simulink model "FaceDetectResponseApp"  (R2023a)
settings: Solver=FixedStepAuto  StartTime=0.0  StopTime=inf  RelTol=1e-3
undefined symbols (not defined in the file): Rec, SDTV
libraries: androiduilib x6, visionconversions x3, androidaudiovideolib x2, visiontextngfix x2, androidcommunicationlib x1
settings Model: Creator=The MathWorks, Inc.  LastModifiedBy=aqeel
settings SolverCC: AlgebraicLoopSolver=TrustRegion
settings DataIOCC: ReturnWorkspaceOutputs=off
settings OptimizationCC: EnhancedBackFolding=on  PassReuseOutputArgsAs=Individual arguments  ZeroExternalMemoryAtStartup=off  ZeroInternalMemoryAtStartup=off  MaxStackSize=64  OptimizeBlockOrder=speed  DifferentSizesBufferReuse=on  OptimizationCustomize=off  EfficientTunableParamExpr=on
settings DebuggingCC: ParameterTunabilityLossMsg=error  UnconnectedInputMsg=warning  UnconnectedOutputMsg=warning  UnconnectedLineMsg=warning  ArithmeticOperatorsInVariantConditions=warning
settings HardwareCC: ProdBitPerPointer=32  ProdBitPerSizeT=32  ProdBitPerPtrDiffT=32  ProdLargestAtomicInteger=Long  ProdLargestAtomicFloat=Double  ProdWordSize=32  ProdHWDeviceType=ARM Compatible->ARM Cortex  UseEmbeddedCoderFeatures=off  UseSimulinkCoderFeatures=off
settings ModelReferenceCC: EnableRefExpFcnMdlSchedulingChecks=on
settings SFSimCC: CustomCodeUndefinedFunction=UseInterfaceOnly
settings RTWCC: Description=Embedded Coder  SystemTargetFile=ert.tlc  HardwareBoard=Android Device  TLCOptions="-aInlineSetEventsForThisBaseRateFcn=TLC_FALSE -aSuppressMultiTaskScheduler=TLC_FALSE  -aRateBasedStepFcn=0"  TemplateMakefile=ert_default_tmf  GenerateReport=on  RTWVerbose=off  Toolchain=Android SDK/NDK Tools  LaunchReport=on  DLArmComputeVersion=19.05
settings CodeAppCC: ForceParamTrailComments=on  IgnoreCustomStorageClasses=off  OperatorAnnotations=on  SimulinkDataObjDesc=on  SFDataObjDesc=on  InsertBlockDesc=on
settings ERTTargetCC: SupportNonInlinedSFcns=on

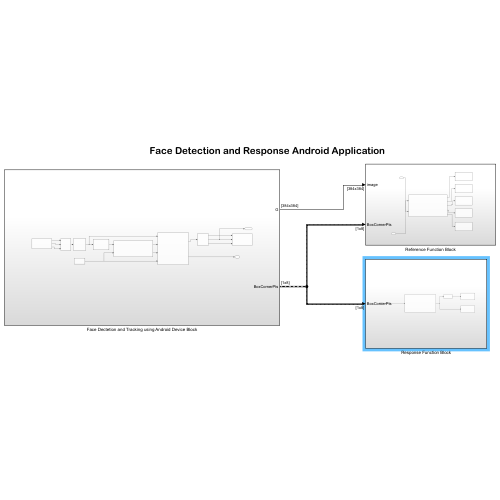
[thumbnail: Simulink's stored preview of the top-level diagram]
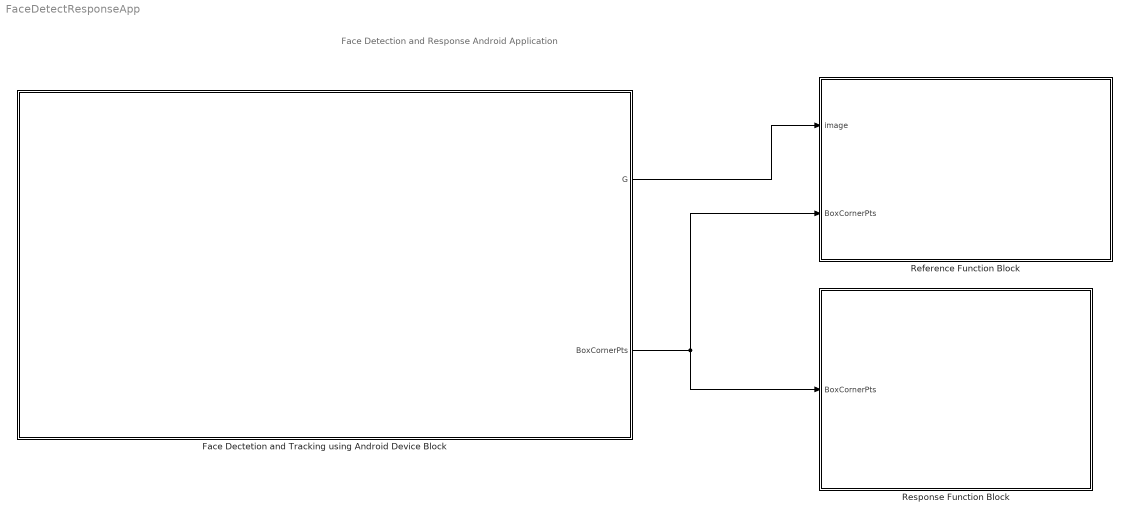
== system FaceDetectResponseApp ==
  note: Face Detection and Response Android Application
  Face Dectetion and Tracking using Android Device Block : Subsystem
  Reference Function Block : Subsystem
  Response Function Block : Subsystem
  wires:
  Face Dectetion and Tracking using Android Device Block/2(BoxCornerPts) -> Response Function Block/1(BoxCornerPts), Reference Function Block/2(BoxCornerPts)
  Face Dectetion and Tracking using Android Device Block/1(G) -> Reference Function Block/1(image)

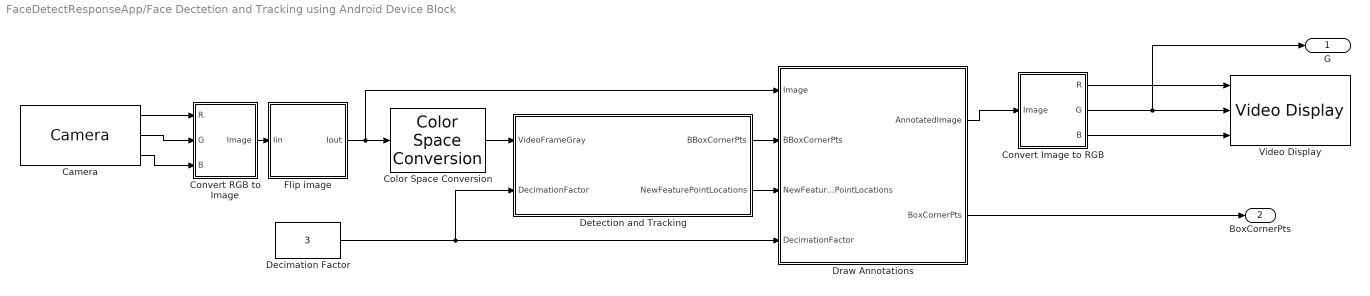
== system FaceDetectResponseApp/Face Dectetion and Tracking using Android Device Block ==
  Camera : androidaudiovideolib/Camera  CameraLocation=Back  CameraResolutions=Back - 384x384  Width=384  Height=384  SampleTime=0.01  BlockPlatform=Android
  Color Space Conversion : visionconversions/Color Space  Conversion  conversion=Obsolete  conversionActive=R'G'B' to intensity  wp_str=D65  rec=Rec. 601 (SDTV)  sys=1125/60/2:1  imagePorts=One multidimensional signal
  Convert Image to RGB : Subsystem
  Convert RGB to Image : Subsystem
  Decimation Factor : Constant  Value=3
  Detection and Tracking : Subsystem
  Draw Annotations : Subsystem
  Flip image : MATLAB Function  TreatAsAtomicUnit=on
  Video Display : androidaudiovideolib/Video Display  BlockPlatform=Android
  G : Outport
  BoxCornerPts : Outport  Port=2
  wires:
  Draw Annotations/2(BoxCornerPts) -> BoxCornerPts/1
  Flip image/1(Iout) -> Draw Annotations/1(Image), Color Space Conversion/1
  Detection and Tracking/1(BBoxCornerPts) -> Draw Annotations/2(BBoxCornerPts)
  Decimation Factor/1 -> Draw Annotations/4(DecimationFactor), Detection and Tracking/2(DecimationFactor)
  Camera/3 -> Convert RGB to Image/3(B)
  Convert Image to RGB/2(G) -> G/1, Video Display/2
  Draw Annotations/1(AnnotatedImage) -> Convert Image to RGB/1(Image)
  Camera/2 -> Convert RGB to Image/2(G)
  Convert Image to RGB/1(R) -> Video Display/1
  Convert RGB to Image/1(Image) -> Flip image/1(Iin)
  Color Space Conversion/1 -> Detection and Tracking/1(VideoFrameGray)
  Detection and Tracking/2(NewFeaturePointLocations) -> Draw Annotations/3(NewFeaturePointLocations)
  Convert Image to RGB/3(B) -> Video Display/3
  Camera/1 -> Convert RGB to Image/1(R)

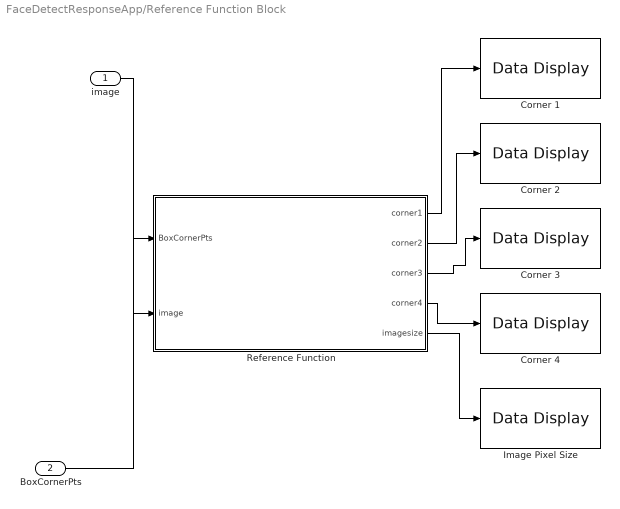
== system FaceDetectResponseApp/Reference Function Block ==
  image : Inport
  BoxCornerPts : Inport  Port=2
  Corner 1 : androiduilib/Data Display  DataDisplayId=FaceDetectResponseApp/Reference_Function_Block/Corner_1  Format=Integer  Precision=6  SimulateUsing=Code generation  blockPlatform=Android
  Corner 2 : androiduilib/Data Display  DataDisplayId=FaceDetectResponseApp/Reference_Function_Block/Corner_2  Format=Integer  Precision=6  SimulateUsing=Code generation  blockPlatform=Android
  Corner 3 : androiduilib/Data Display  DataDisplayId=FaceDetectResponseApp/Reference_Function_Block/Corner_3  Format=Integer  Precision=6  SimulateUsing=Code generation  blockPlatform=Android
  Corner 4 : androiduilib/Data Display  DataDisplayId=FaceDetectResponseApp/Reference_Function_Block/Corner_4  Format=Integer  Precision=6  SimulateUsing=Code generation  blockPlatform=Android
  Image Pixel Size : androiduilib/Data Display  DataDisplayId=FaceDetectResponseApp/Reference_Function_Block/Image_Pixel_Size  Format=Float  Precision=6  SimulateUsing=Code generation  blockPlatform=Android
  Reference Function : MATLAB Function  TreatAsAtomicUnit=on
  wires:
  Reference Function/2(corner2) -> Corner 2/1
  Reference Function/4(corner4) -> Corner 4/1
  Reference Function/3(corner3) -> Corner 3/1
  Reference Function/1(corner1) -> Corner 1/1
  BoxCornerPts/1 -> Reference Function/1(BoxCornerPts)
  Reference Function/5(imagesize) -> Image Pixel Size/1
  image/1 -> Reference Function/2(image)

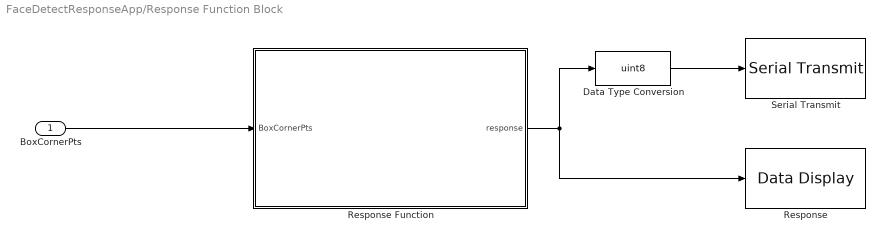
== system FaceDetectResponseApp/Response Function Block ==
  BoxCornerPts : Inport
  Data Type Conversion : DataTypeConversion  OutDataTypeStr=uint8  SaturateOnIntegerOverflow=off  RndMeth=Floor
  Response : androiduilib/Data Display  DataDisplayId=FaceDetectResponseApp/Response_Function_Block/Response  Format=Integer  Precision=6  SimulateUsing=Code generation  blockPlatform=Android
  Response Function : MATLAB Function  TreatAsAtomicUnit=on
  Serial Transmit : androidcommunicationlib/Serial Transmit
  wires:
  Data Type Conversion/1 -> Serial Transmit/1
  Response Function/1(response) -> Response/1, Data Type Conversion/1
  BoxCornerPts/1 -> Response Function/1(BoxCornerPts)

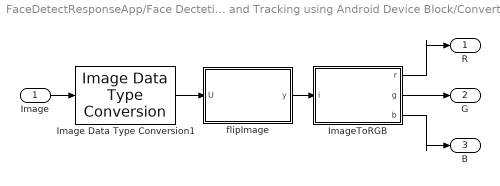
== system FaceDetectResponseApp/Face Dectetion and Tracking using Android Device Block/Convert Image to RGB ==
  Image : Inport
  Image Data Type Conversion1 : visionconversions/Image Data Type Conversion  outDT=uint8  isSigned=on  wordLen=16  numFracBits=0
  ImageToRGB : MATLAB Function  TreatAsAtomicUnit=on
  flipImage : MATLAB Function  TreatAsAtomicUnit=on
  R : Outport
  G : Outport  Port=2
  B : Outport  Port=3
  wires:
  ImageToRGB/3(b) -> B/1
  flipImage/1(y) -> ImageToRGB/1(i)
  Image Data Type Conversion1/1 -> flipImage/1(U)
  ImageToRGB/2(g) -> G/1
  ImageToRGB/1(r) -> R/1
  Image/1 -> Image Data Type Conversion1/1

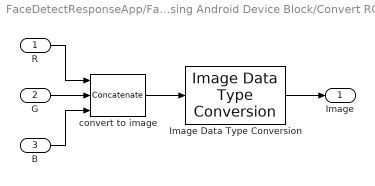
== system FaceDetectResponseApp/Face Dectetion and Tracking using Android Device Block/Convert RGB to Image ==
  R : Inport
  G : Inport  Port=2
  B : Inport  Port=3
  Image Data Type Conversion : visionconversions/Image Data Type Conversion  outDT=single  isSigned=on  wordLen=16  numFracBits=0
  convert to image : Concatenate  NumInputs=3  Mode=Multidimensional array  ConcatenateDimension=3
  Image : Outport
  wires:
  convert to image/1 -> Image Data Type Conversion/1
  B/1 -> convert to image/3
  G/1 -> convert to image/2
  R/1 -> convert to image/1
  Image Data Type Conversion/1 -> Image/1

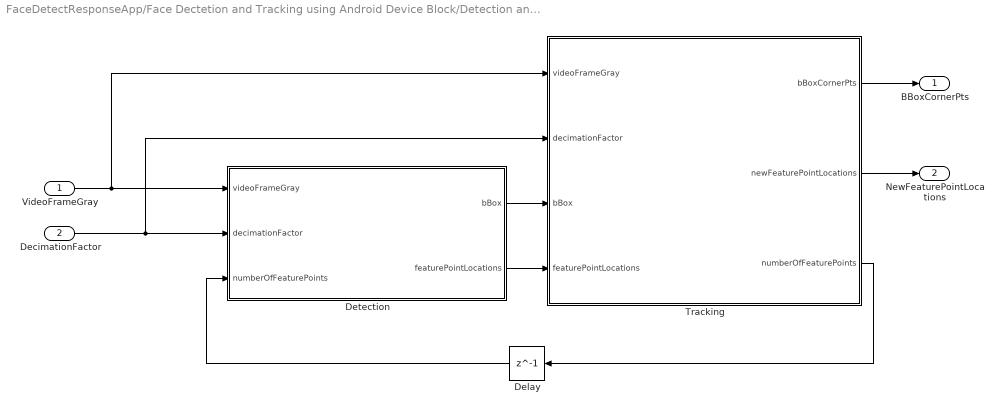
== system FaceDetectResponseApp/Face Dectetion and Tracking using Android Device Block/Detection and Tracking ==
  VideoFrameGray : Inport
  DecimationFactor : Inport  Port=2
  Delay : Delay  DelayLength=1
  Detection : MATLAB Function  TreatAsAtomicUnit=on
  Tracking : MATLAB Function  TreatAsAtomicUnit=on
  BBoxCornerPts : Outport  VectorParamsAs1DForOutWhenUnconnected=off
  NewFeaturePointLocations : Outport  Port=2  VectorParamsAs1DForOutWhenUnconnected=off
  wires:
  VideoFrameGray/1 -> Tracking/1(videoFrameGray), Detection/1(videoFrameGray)
  Detection/1(bBox) -> Tracking/3(bBox)
  Detection/2(featurePointLocations) -> Tracking/4(featurePointLocations)
  Tracking/1(bBoxCornerPts) -> BBoxCornerPts/1
  Tracking/2(newFeaturePointLocations) -> NewFeaturePointLocations/1
  DecimationFactor/1 -> Tracking/2(decimationFactor), Detection/2(decimationFactor)
  Tracking/3(numberOfFeaturePoints) -> Delay/1
  Delay/1 -> Detection/3(numberOfFeaturePoints)

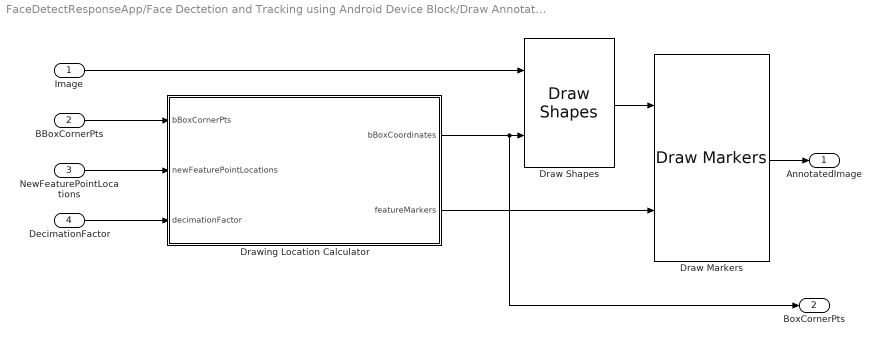
== system FaceDetectResponseApp/Face Dectetion and Tracking using Android Device Block/Draw Annotations ==
  Image : Inport
  BBoxCornerPts : Inport  Port=2
  NewFeaturePointLocations : Inport  Port=3
  DecimationFactor : Inport  Port=4
  Draw Markers : visiontextngfix/Draw Markers  shape=Plus  size=3  fill=off  fillClrSource=Specify via dialog  display=White  intensity=200  color=[200 255 100]  opacity=0.6  viewport=Entire image  antialiasing=off  inType=Obsolete  imagePorts=One multidimensional signal  roundingMode=Floor  overflowMode=off  memoryMode=Specify word length  memoryWordLength=16  memoryFracLength=15  prodOutputMode=Binary point scaling  prodOutputWordLength=32  prodOutputFracLength=14
  Draw Shapes : visiontextngfix/Draw Shapes  shape=Polygons  fill=off  lineWidth=1  fillClrSource=Specify via dialog  display=User-specified value  intensity=200  color=[255 255 0]  opacity=0.6  viewport=Entire image  antialiasing=off  inType=Obsolete  imagePorts=One multidimensional signal  roundingMode=Floor  overflowMode=off  memoryMode=Specify word length  memoryWordLength=16  prodOutputMode=Binary point scaling  prodOutputWordLength=32  prodOutputFracLength=14  memoryFracLength=14
  Drawing Location Calculator : MATLAB Function  TreatAsAtomicUnit=on
  AnnotatedImage : Outport  VectorParamsAs1DForOutWhenUnconnected=off
  BoxCornerPts : Outport  Port=2  VectorParamsAs1DForOutWhenUnconnected=off
  wires:
  Drawing Location Calculator/1(bBoxCoordinates) -> BoxCornerPts/1, Draw Shapes/2
  Draw Markers/1 -> AnnotatedImage/1
  Drawing Location Calculator/2(featureMarkers) -> Draw Markers/2
  Image/1 -> Draw Shapes/1
  BBoxCornerPts/1 -> Drawing Location Calculator/1(bBoxCornerPts)
  NewFeaturePointLocations/1 -> Drawing Location Calculator/2(newFeaturePointLocations)
  Draw Shapes/1 -> Draw Markers/1
  DecimationFactor/1 -> Drawing Location Calculator/3(decimationFactor)

== matlab function FaceDetectResponseApp/Face Dectetion and Tracking using Android Device Block/Detection and Tracking/Tracking ==
  data: videoFrameGray input; decimationFactor input; bBox input size=[2 8]; bBoxCornerPts output size=[4 2]; featurePointLocations input size=[500 2]; newFeaturePointLocations output size=[500 2]; numberOfFeaturePoints output
% Function for tracking face and feature points
%
% Copyright 2016 The MathWorks, Inc.
function [bBoxCornerPts, newFeaturePointLocations, numberOfFeaturePoints]  = trackPoints(videoFrameGray, decimationFactor, bBox, featurePointLocations)
%#codegen
persistent pointTracker
persistent oldPoints
persistent bboxPoints
persistent first_time
persistent numPts

% Create the point tracker object.
if isempty(pointTracker)
    pointTracker = vision.PointTracker('MaxBidirectionalError', 2);
end

if isempty(bboxPoints)
    bboxPoints = [0 0];
end 

if isempty(oldPoints)
    oldPoints = single([0 0]);
end      

if isempty(numPts)
    numPts = 0;
end

% Resize frame
videoFrameGray = videoFrameGray(1:decimationFactor:end,1:decimationFactor:end);

% Initialize tracker with dummy points
if isempty(first_time)
   initialize(pointTracker, single([10 10]), videoFrameGray);
   first_time = 0;
end

if numPts < 10
    if ~isempty(featurePointLocations)
        % Re-initialize the point tracker if a face has been detected and
        % feature points obtained.
        newFeaturePointLocations = featurePointLocations;
        numPts = size(newFeaturePointLocations,1);
        
        if ~pointTracker.isLocked
            initialize(pointTracker, newFeaturePointLocations, videoFrameGray);
        end
        step(pointTracker, videoFrameGray);
        setPoints(pointTracker, newFeaturePointLocations);
        
        % Save a copy of the points.
        oldPoints = newFeaturePointLocations;
        
        % Convert the rectangle represented as [x, y, w, h] into an
        % M-by-2 matrix of [x,y] coordinates of the four corners. This
        % is needed to be able to transform the bounding box to display
        % the orientation of the face.
        bboxPoints = bbox2points(bBox(1, :));
        bBoxCornerPts = bboxPoints;
    else
        bBoxCornerPts = [];
        newFeaturePointLocations = single([]);
    end

else
    % Tracking mode. 
    [newFeaturePointLocations, isFound] = step(pointTracker, videoFrameGray);
    assert(size(newFeaturePointLocations, 1) < 500);
    visiblePoints = newFeaturePointLocations(isFound, :);
    oldInliers = oldPoints(isFound, :);

    numPts = size(visiblePoints, 1);

    if numPts >= 10
        % Estimate the geometric transformation between the old points
        % and the new points.
        [xform, inlierIdx] = estimateGeometricTransform2D(...
            oldInliers, visiblePoints, 'similarity', 'MaxDistance', 4);
        visiblePoints = visiblePoints(inlierIdx, :);

        % Apply the transformation to the bounding box.
        bboxPoints = double(transformPointsForward(xform, bboxPoints));
        bBoxCornerPts = bboxPoints;

        % Assign the visible feature points
        assert(size(visiblePoints, 1) < 500);
        newFeaturePointLocations = visiblePoints;
        
        % Reset the points.
        oldPoints = visiblePoints;
        setPoints(pointTracker, oldPoints);
    else
        bBoxCornerPts = [];
        newFeaturePointLocations = single([]);            
    end

end

numberOfFeaturePoints = numPts;

== matlab function FaceDetectResponseApp/Face Dectetion and Tracking using Android Device Block/Detection and Tracking/Detection ==
  data: bBox output size=[2 8]; videoFrameGray input; featurePointLocations output size=[500 2]; decimationFactor input; numberOfFeaturePoints input
% Function for detecting a face and feature points.
%
% Copyright 2016 The MathWorks, Inc.
function [bBox, featurePointLocations]  = detectFaceAndFeatures(...
    videoFrameGray, decimationFactor, numberOfFeaturePoints)

%#codegen
persistent faceDetector

% Resize frame
videoFrameGray = videoFrameGray(1:decimationFactor:end,1:decimationFactor:end);

% Perform detection when the number of points being tracked goes below a
% certain threshold. These points may be just outliers.
%if numberOfFeaturePoints < 10
    % Detection mode
    
    % Create the face detector object.
    if isempty(faceDetector)
        faceDetector = vision.CascadeObjectDetector('/sdcard/haarcascade_frontalface_alt2.xml');
    end

    bBox = faceDetector.step(videoFrameGray);
    % Asser if a face is not detected.
    assert(size(bBox, 1) < 10);
    
    if ~isempty(bBox)
        % Find corner points inside the detected region.
        points = detectMinEigenFeatures(videoFrameGray, 'ROI', bBox(1, :));    
        featurePointLocations = points.Location;
    else
        % Return emtpty if no face detected.
        featurePointLocations = single([]);
    end
% else
%     % Return empty if once face is detected and valid.
%     bBox = [];
%     featurePointLocations = single([]);
% end

== matlab function FaceDetectResponseApp/Face Dectetion and Tracking using Android Device Block/Draw Annotations/Drawing Location Calculator ==
  data: bBoxCornerPts input size=[4 2]; bBoxCoordinates output size=[1 8]; newFeaturePointLocations input size=[500 2]; featureMarkers output size=[500 2]; decimationFactor input
% Function for calculating drawing locations
%
% Copyright 2016 The MathWorks, Inc.
function [bBoxCoordinates, featureMarkers]  = obtainDrawingLocations(bBoxCornerPts, newFeaturePointLocations, decimationFactor)

if ~isempty(bBoxCornerPts)
    % Convert the box corners into the [x1 y1 x2 y2 x3 y3 x4 y4]
    % format required by insertShape.
    bboxPolygon = reshape(bBoxCornerPts', 1, []);
    
    % Display a bounding box around the detected face.
    bBoxCoordinates = bboxPolygon.* decimationFactor;
   
    % Display detected corners.
    featureMarkers = newFeaturePointLocations.* decimationFactor;
else
    % Draw Markers and Draw Shapes block expect an input to be provided.
    % Hence providing the following input when nothing to be drawn.
    bBoxCoordinates = [0 0 0 0 0 0 0 0];
    featureMarkers = single([0 0]);
end

== matlab function FaceDetectResponseApp/Face Dectetion and Tracking using Android Device Block/Convert Image to RGB/ImageToRGB ==
  data: i input; r output; g output; b output
function [r, g, b] = ImageToRGB(i)
r=i(:,:,1);
g=i(:,:,2);
b=i(:,:,3);

== matlab function FaceDetectResponseApp/Face Dectetion and Tracking using Android Device Block/Flip image ==
  data: Iin input; Iout output
function Iout = flip(Iin)
%rotate image anti clockwise 90 degrees
Iin= imrotate( Iin , 90 );
%Flip image
Iin=flipdim(Iin,1);
Iout = Iin;

== matlab function FaceDetectResponseApp/Face Dectetion and Tracking using Android Device Block/Convert Image to RGB/flipImage ==
  data: U input; y output
function y = flipImage(U)
U= imrotate( U , 90 );
%Flip image
U=flipdim(U,1);

y = U;

== matlab function FaceDetectResponseApp/Reference Function Block/Reference Function ==
  data: BoxCornerPts input size=[1 8]; corner1 output size=[1 2]; corner2 output size=[1 2]; corner3 output size=[1 2]; corner4 output size=[1 2]; image input; imagesize output
% Function to show the coordinates of each corner on the android device for
% reference.

function [corner1,corner2,corner3,corner4,imagesize]   = ReferenceFunction(BoxCornerPts,image)

corner1 = [BoxCornerPts(1,1) BoxCornerPts(1,2)];
corner2 = [BoxCornerPts(1,3) BoxCornerPts(1,4)];
corner3 = [BoxCornerPts(1,5) BoxCornerPts(1,6)];
corner4 = [BoxCornerPts(1,7) BoxCornerPts(1,8)];
imagesize = size(image);
end

== matlab function FaceDetectResponseApp/Response Function Block/Response Function ==
  data: BoxCornerPts input size=[1 8]; response output size=1
% Function to use corner points from the face detection to determine what
% repsonse is required to move the arduino robot to achieve the required
% distance between robot and detected face.

%Robot Controls:
%response = 0 --> Stop
%response = 1 --> Forward
%response = 2 --> Reverse
%response = 3 --> Right
%response = 4 --> Left

function response  = ResponseFunction(BoxCornerPts)

if sum(BoxCornerPts)==0 %If no face is detected, there would be no points in matrix.
    response = 0;
else
    corner1 = [BoxCornerPts(1) BoxCornerPts(2)];
    corner3 = [BoxCornerPts(5) BoxCornerPts(6)];
    point1 = (corner1+corner3)/2; %Mid Point of Box
    point2 = [192 192]; %Mid Point of Image (This should be  changed based on pixel size)
    area = ((corner1(1)-corner3(1))^2+(corner1(2)-corner3(2))^2)/2;
    if area > 128*128 %Approximate size of the maximum box, assume a third of image size.
        response = 0;
        if area > 256*256 %Approximate maximum size of box if too close.
            response=2;
        end
    else 
        if point1(1)-point2(1)<-60 %Maximum difference to initiate a left turn (dependent on image size)
            response = 4;
        else 
            if point1(1)-point2(1)>60 %Maximum difference to initiate a right turn (dependent on image size)
                response = 3;
            else 
                response = 1;
            end
        end
    end
end
end
